simulink model "simulink_stato_scalare"  (R2024a)
settings: Solver=FixedStepAuto  StartTime=0.0  StopTime=T_max  FixedStep=ST  RelTol=1e-3
values from neighbouring files (symbols this model uses):
  a_m = 1    [init.m]
  a_r = 1.1    [init.m]
  alfa = 1    [init.m]
  b_m = 1    [init.m]
  centri_f = zeros(1,numero_nodi_f)    [init.m]
  centri_H = zeros(1,numero_nodi_H)    [init.m]
  k_m = 10    [init.m]
  k_r = 10    [init.m]
  lr_f = 0.2    [init.m]
  lr_H = 1    [init.m]
  M_f = 100    [init.m]
  M_H = 0.5    [init.m]
  numero_nodi_f = 41    [init.m]
  numero_nodi_H = 41    [init.m]
  omega_r = 5*2*pi/T_max    (= 0.261799387799)    [init.m]
  q_init = 0    [init.m]
  q_limit = pi    (= 3.14159265359)    [init.m]
  var_f = delta_q_f^2/2/log(2)    [init.m]
  var_H = delta_q_H^2/2/log(2)    [init.m]
settings Model: Creator=gabri  LastModifiedBy=gabri

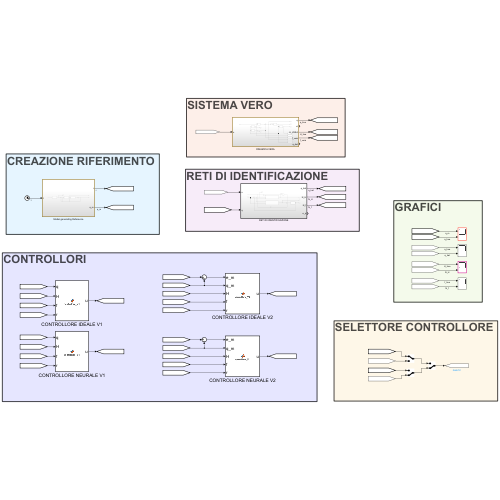
[thumbnail: Simulink's stored preview of the top-level diagram]
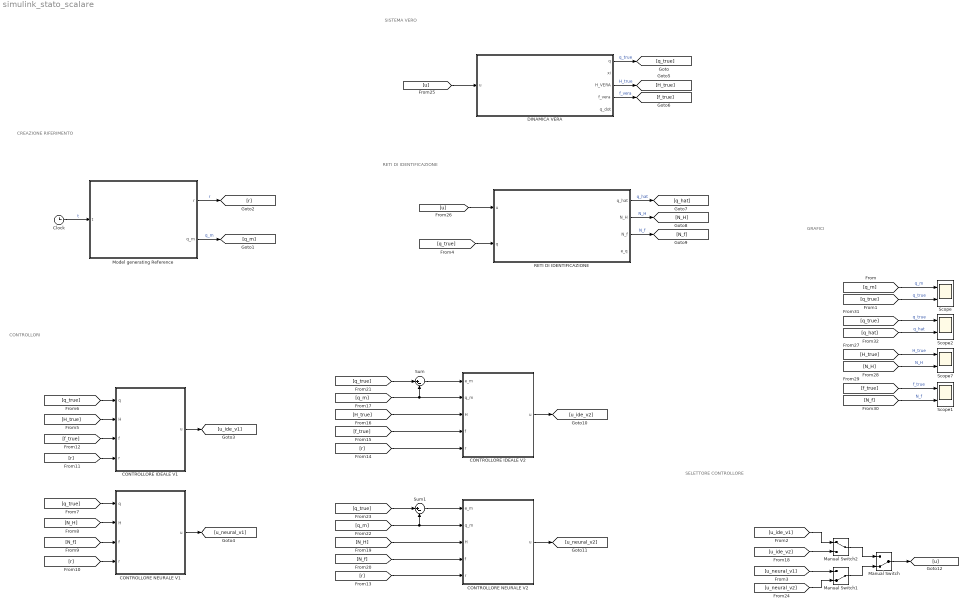
== system simulink_stato_scalare ==
  note: CREAZIONE RIFERIMENTO
  note: RETI DI IDENTIFICAZIONE
  note: SISTEMA VERO
  note: GRAFICI
  note: SELETTORE CONTROLLORE
  note: CONTROLLORI
  CONTROLLORE IDEALE V1 : MATLAB Function  TreatAsAtomicUnit=on
  CONTROLLORE IDEALE V2 : MATLAB Function  TreatAsAtomicUnit=on
  CONTROLLORE NEURALE V1 : MATLAB Function  TreatAsAtomicUnit=on
  CONTROLLORE NEURALE V2 : MATLAB Function  TreatAsAtomicUnit=on
  Clock : Clock
  DINAMICA VERA : Subsystem
  Manual Switch : ManualSwitch  CurrentSetting=0
  Manual Switch1 : ManualSwitch  CurrentSetting=0
  Manual Switch2 : ManualSwitch
  Model generating Reference : Subsystem
  RETI DI IDENTIFICAZIONE : Subsystem
  Scope{,1..2,7} (4 alike) : Scope  NumInputPorts=2
  Sum : Sum  Inputs=|+-
  Sum1 : Sum  Inputs=|+-
  wires:
  Clock/1 -> Model generating Reference/1(t)  "t"
  Model generating Reference/2(q_m) -> [q_m]  "q_m"
  [q_m] -> Scope/1  "q_m"
  [q_true] -> Scope/2  "q_true"
  Model generating Reference/1(r) -> [r]  "r"
  CONTROLLORE IDEALE V1/1(u) -> [u_ide_v1]
  CONTROLLORE NEURALE V1/1(u) -> [u_neural_v1]
  DINAMICA VERA/1(q) -> [q_true]  "q_true"
  DINAMICA VERA/3(H_VERA) -> [H_true]  "H_true"
  DINAMICA VERA/4(f_vera) -> [f_true]  "f_vera"
  Manual Switch1/1 -> Manual Switch/2
  Manual Switch2/1 -> Manual Switch/1
  [u_ide_v1] -> Manual Switch2/1
  [u_neural_v1] -> Manual Switch1/1
  [q_true] -> RETI DI IDENTIFICAZIONE/2(q)
  RETI DI IDENTIFICAZIONE/1(q_hat) -> [q_hat]  "q_hat"
  RETI DI IDENTIFICAZIONE/2(N_H) -> [N_H]  "N_H"
  RETI DI IDENTIFICAZIONE/3(N_f) -> [N_f]  "N_f"
  [H_true] -> CONTROLLORE IDEALE V1/2(H)
  [q_true] -> CONTROLLORE IDEALE V1/1(q)
  [q_true] -> CONTROLLORE NEURALE V1/1(q)
  [N_H] -> CONTROLLORE NEURALE V1/2(H)
  [N_f] -> CONTROLLORE NEURALE V1/3(f)
  [r] -> CONTROLLORE NEURALE V1/4(r)
  [r] -> CONTROLLORE IDEALE V1/4(r)
  [f_true] -> CONTROLLORE IDEALE V1/3(f)
  [f_true] -> CONTROLLORE IDEALE V2/4(f)
  [r] -> CONTROLLORE IDEALE V2/5(r)
  [r] -> CONTROLLORE NEURALE V2/5(r)
  [N_f] -> CONTROLLORE NEURALE V2/4(f)
  [N_H] -> CONTROLLORE NEURALE V2/3(H)
  [q_m] -> Sum/2, CONTROLLORE IDEALE V2/2(q_m)
  [H_true] -> CONTROLLORE IDEALE V2/3(H)
  [q_true] -> Sum/1
  Sum/1 -> CONTROLLORE IDEALE V2/1(e_m)
  Sum1/1 -> CONTROLLORE NEURALE V2/1(e_m)
  [q_true] -> Sum1/1
  [q_m] -> CONTROLLORE NEURALE V2/2(q_m), Sum1/2
  CONTROLLORE NEURALE V2/1(u) -> [u_neural_v2]
  CONTROLLORE IDEALE V2/1(u) -> [u_ide_v2]
  [u_neural_v2] -> Manual Switch1/2
  [u_ide_v2] -> Manual Switch2/2
  Manual Switch/1 -> [u]
  [u] -> DINAMICA VERA/1(u)
  [u] -> RETI DI IDENTIFICAZIONE/1(u)
  [H_true] -> Scope7/1  "H_true"
  [N_H] -> Scope7/2  "N_H"
  [N_f] -> Scope1/2  "N_f"
  [f_true] -> Scope1/1  "f_true"
  [q_hat] -> Scope2/2  "q_hat"
  [q_true] -> Scope2/1  "q_true"

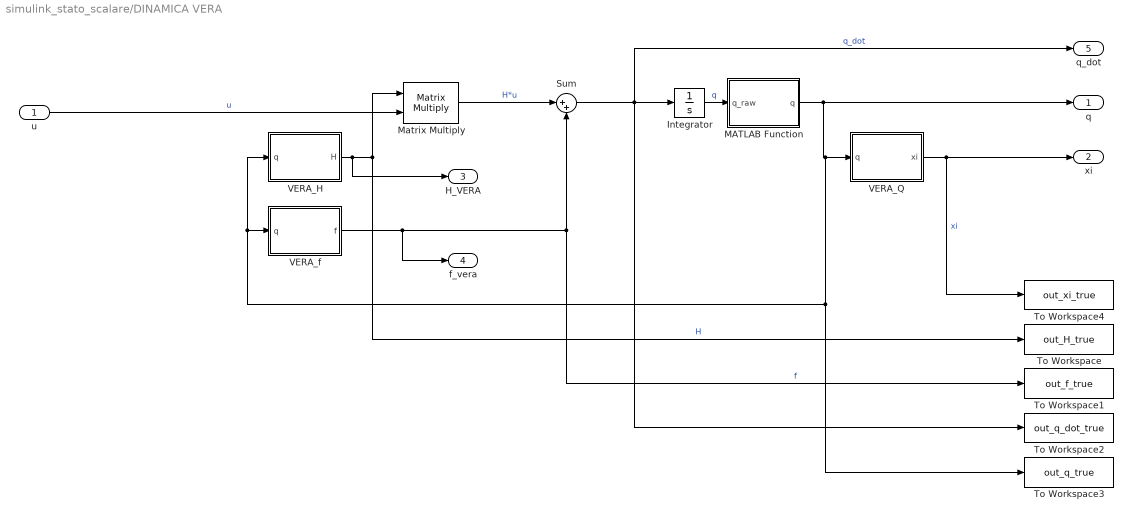
== system simulink_stato_scalare/DINAMICA VERA ==
  u : Inport
  Integrator : Integrator  InitialCondition=q_init
  MATLAB Function : MATLAB Function  TreatAsAtomicUnit=on
  Matrix Multiply : Product  Multiplication=Matrix(*)
  Sum : Sum  Inputs=|++
  To Workspace : ToWorkspace  VariableName=out_H_true  SaveFormat=Timeseries  SampleTime=-1
  To Workspace1 : ToWorkspace  VariableName=out_f_true  SaveFormat=Timeseries  SampleTime=-1
  To Workspace2 : ToWorkspace  VariableName=out_q_dot_true  SaveFormat=Timeseries  SampleTime=-1
  To Workspace3 : ToWorkspace  VariableName=out_q_true  SaveFormat=Timeseries  SampleTime=-1
  To Workspace4 : ToWorkspace  VariableName=out_xi_true  SaveFormat=Timeseries  SampleTime=-1
  VERA_H : MATLAB Function  TreatAsAtomicUnit=on
  VERA_Q : MATLAB Function  TreatAsAtomicUnit=on
  VERA_f : MATLAB Function  TreatAsAtomicUnit=on
  q : Outport
  xi : Outport  Port=2
  H_VERA : Outport  Port=3
  f_vera : Outport  Port=4
  q_dot : Outport  Port=5
  wires:
  VERA_H/1(H) -> H_VERA/1, To Workspace/1, Matrix Multiply/1  "H"
  u/1 -> Matrix Multiply/2  "u"
  Matrix Multiply/1 -> Sum/1  "H*u"
  VERA_f/1(f) -> f_vera/1, To Workspace1/1, Sum/2  "f"
  Sum/1 -> q_dot/1, To Workspace2/1, Integrator/1  "q_dot"
  VERA_Q/1(xi) -> To Workspace4/1, xi/1  "xi"
  Integrator/1 -> MATLAB Function/1(q_raw)  "q"
  MATLAB Function/1(q) -> VERA_H/1(q), VERA_f/1(q), To Workspace3/1, VERA_Q/1(q), q/1

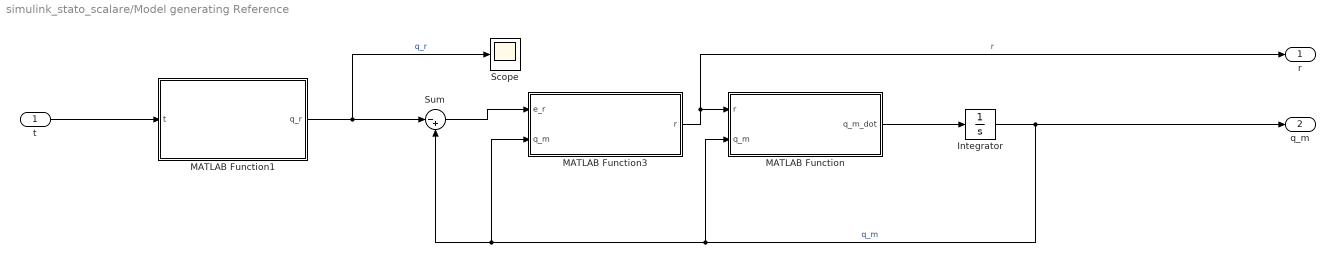
== system simulink_stato_scalare/Model generating Reference ==
  t : Inport
  Integrator : Integrator
  MATLAB Function : MATLAB Function  TreatAsAtomicUnit=on
  MATLAB Function1 : MATLAB Function  TreatAsAtomicUnit=on
  MATLAB Function3 : MATLAB Function  TreatAsAtomicUnit=on
  Scope : Scope
  Sum : Sum  Inputs=|-+
  r : Outport
  q_m : Outport  Port=2
  wires:
  MATLAB Function1/1(q_r) -> Sum/1, Scope/1  "q_r"
  Integrator/1 -> q_m/1, MATLAB Function3/2(q_m), Sum/2, MATLAB Function/2(q_m)  "q_m"
  t/1 -> MATLAB Function1/1(t)
  MATLAB Function3/1(r) -> r/1, MATLAB Function/1(r)  "r"
  MATLAB Function/1(q_m_dot) -> Integrator/1
  Sum/1 -> MATLAB Function3/1(e_r)

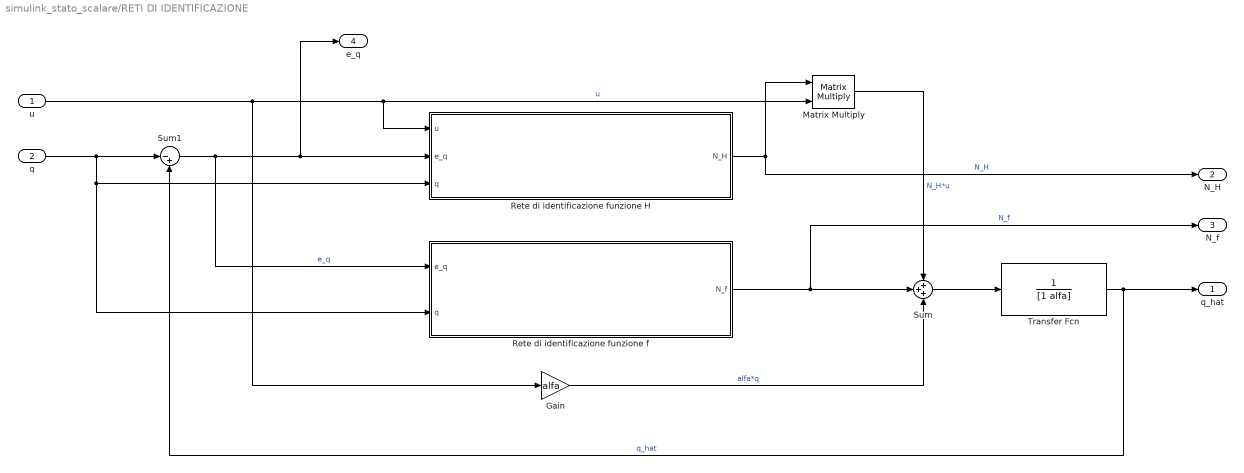
== system simulink_stato_scalare/RETI DI IDENTIFICAZIONE ==
  u : Inport
  q : Inport  Port=2
  Gain : Gain  Gain=alfa
  Matrix Multiply : Product  Multiplication=Matrix(*)
  Rete di identificazione funzione H : Subsystem
  Rete di identificazione funzione f : Subsystem
  Sum : Sum  Inputs=+++
  Sum1 : Sum  Inputs=|-+
  Transfer Fcn : TransferFcn  Denominator=[1 alfa]
  q_hat : Outport
  N_H : Outport  Port=2
  N_f : Outport  Port=3
  e_q : Outport  Port=4
  wires:
  u/1 -> Gain/1, Rete di identificazione funzione H/1(u), Matrix Multiply/2  "u"
  Rete di identificazione funzione H/1(N_H) -> N_H/1, Matrix Multiply/1  "N_H"
  Matrix Multiply/1 -> Sum/1  "N_H*u"
  q/1 -> Sum1/1, Rete di identificazione funzione f/2(q), Rete di identificazione funzione H/3(q)
  Rete di identificazione funzione f/1(N_f) -> N_f/1, Sum/2  "N_f"
  Sum/1 -> Transfer Fcn/1
  Transfer Fcn/1 -> Sum1/2, q_hat/1  "q_hat"
  Gain/1 -> Sum/3  "alfa*q"
  Sum1/1 -> Rete di identificazione funzione f/1(e_q), e_q/1, Rete di identificazione funzione H/2(e_q)  "e_q"

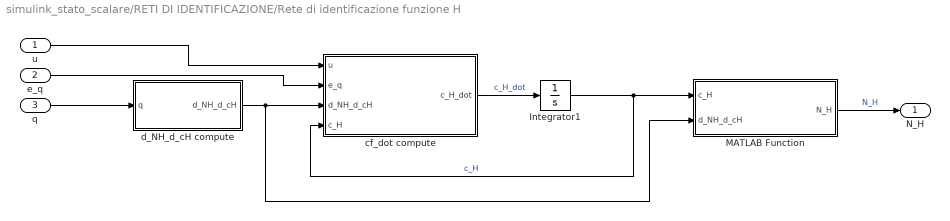
== system simulink_stato_scalare/RETI DI IDENTIFICAZIONE/Rete di identificazione funzione H ==
  u : Inport
  e_q : Inport  Port=2
  q : Inport  Port=3
  Integrator1 : Integrator  InitialCondition=c_H_init'
  MATLAB Function : MATLAB Function  TreatAsAtomicUnit=on
  cf_dot compute : MATLAB Function  TreatAsAtomicUnit=on
  d_NH_d_cH compute : MATLAB Function  TreatAsAtomicUnit=on
  N_H : Outport
  wires:
  MATLAB Function/1(N_H) -> N_H/1  "N_H"
  q/1 -> d_NH_d_cH compute/1(q)
  d_NH_d_cH compute/1(d_NH_d_cH) -> MATLAB Function/2(d_NH_d_cH), cf_dot compute/3(d_NH_d_cH)
  cf_dot compute/1(c_H_dot) -> Integrator1/1  "c_H_dot"
  Integrator1/1 -> MATLAB Function/1(c_H), cf_dot compute/4(c_H)  "c_H"
  e_q/1 -> cf_dot compute/2(e_q)
  u/1 -> cf_dot compute/1(u)

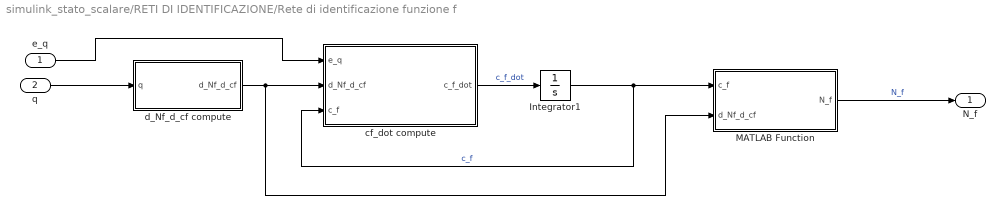
== system simulink_stato_scalare/RETI DI IDENTIFICAZIONE/Rete di identificazione funzione f ==
  e_q : Inport
  q : Inport  Port=2
  Integrator1 : Integrator  InitialCondition=c_f_init'
  MATLAB Function : MATLAB Function  TreatAsAtomicUnit=on
  cf_dot compute : MATLAB Function  TreatAsAtomicUnit=on
  d_Nf_d_cf compute : MATLAB Function  TreatAsAtomicUnit=on
  N_f : Outport
  wires:
  e_q/1 -> cf_dot compute/1(e_q)
  Integrator1/1 -> MATLAB Function/1(c_f), cf_dot compute/3(c_f)  "c_f"
  cf_dot compute/1(c_f_dot) -> Integrator1/1  "c_f_dot"
  d_Nf_d_cf compute/1(d_Nf_d_cf) -> MATLAB Function/2(d_Nf_d_cf), cf_dot compute/2(d_Nf_d_cf)
  q/1 -> d_Nf_d_cf compute/1(q)
  MATLAB Function/1(N_f) -> N_f/1  "N_f"

== matlab function simulink_stato_scalare/Model generating Reference/MATLAB Function ==
  data: r input; q_m_dot output; q_m input; b_m parameter; a_m parameter
function q_m_dot = reference_dynamic(r, q_m, b_m, a_m)

q_m_dot = -a_m*q_m + b_m*r;

== matlab function simulink_stato_scalare/Model generating Reference/MATLAB Function3 ==
  data: e_r input; r output; q_m input; k_r parameter; b_m parameter; a_m parameter
function r = reference_controller(e_r, q_m, k_r, b_m, a_m)

r = (1/b_m)*(a_m*q_m - k_r*e_r);

== matlab function simulink_stato_scalare/CONTROLLORE IDEALE V1 ==
  data: q input; H input; u output; f input; r input; b_m parameter; a_m parameter
function u = controllore_V1(q, H, f, r, b_m, a_m)

u = (1/H)*(-a_m*q + b_m*r - f);

== matlab function simulink_stato_scalare/CONTROLLORE IDEALE V2 ==
  data: e_m input; q_m input; H input; u output; f input; r input; b_m parameter; a_m parameter; k_m parameter
function u = controllore_V2(e_m, q_m, H, f, r, b_m, a_m, k_m)

u = (1/H)*(-a_m*q_m + b_m*r - f -k_m*e_m);

== matlab function simulink_stato_scalare/DINAMICA VERA/VERA_f ==
  data: q input; f output
function f = f(q)

f = (1/2/pi)*sin(2*pi*q);
% f = -q;

== matlab function simulink_stato_scalare/CONTROLLORE NEURALE V2 ==
  data: e_m input; q_m input; H input; u output; f input; r input; b_m parameter; a_m parameter; k_m parameter
function u = controllore_V2(e_m, q_m, H, f, r, b_m, a_m, k_m)

u = (1/H)*(-a_m*q_m + b_m*r - f -k_m*e_m);

== matlab function simulink_stato_scalare/RETI DI IDENTIFICAZIONE/Rete di identificazione funzione H/cf_dot compute ==
  data: u input; e_q input; c_H_dot output; d_NH_d_cH input; M_H parameter; lr_H parameter; c_H input
function c_H_dot = cH_dot(u, e_q, d_NH_d_cH, M_H, lr_H, c_H)

norm_c_H = norm(c_H);

if norm_c_H <= M_H
    c_H_dot = - lr_H * d_NH_d_cH * e_q * u;
else
    c_H_dot = - lr_H * d_NH_d_cH * e_q * u + (lr_H*e_q*c_H'*d_NH_d_cH*u/norm_c_H^2)*c_H;
end

== matlab function simulink_stato_scalare/RETI DI IDENTIFICAZIONE/Rete di identificazione funzione H/d_NH_d_cH compute ==
  data: q input; d_NH_d_cH output; var_H parameter; centri_H parameter; numero_nodi_H parameter
function d_NH_d_cH = d_NH_d_cH(q, var_H, centri_H, numero_nodi_H)

d_NH_d_cH = zeros(numero_nodi_H, 1);

for i=1:numero_nodi_H
    d_NH_d_cH(i) = gaussiana(centri_H(i), var_H, q);
end

== matlab function simulink_stato_scalare/DINAMICA VERA/VERA_H ==
  data: q input; H output
function H = H(q)

H = 1+(1/5/pi)*cos(5*pi*q);
% H = 1;

== matlab function simulink_stato_scalare/DINAMICA VERA/MATLAB Function ==
  data: q_raw input; q output
function q = wrap_to_pi(q_raw)

q = atan2(sin(q_raw), cos(q_raw));

== matlab function simulink_stato_scalare/DINAMICA VERA/VERA_Q ==
  data: q input; xi output
function xi = Q(q)

xi = 10*cos(q);

== matlab function simulink_stato_scalare/RETI DI IDENTIFICAZIONE/Rete di identificazione funzione f/MATLAB Function ==
  data: c_f input; N_f output; d_Nf_d_cf input
function N_f = N_f(c_f, d_Nf_d_cf)

N_f = c_f'*d_Nf_d_cf;

== matlab function simulink_stato_scalare/RETI DI IDENTIFICAZIONE/Rete di identificazione funzione H/MATLAB Function ==
  data: c_H input; N_H output; d_NH_d_cH input
function N_H = N_H(c_H, d_NH_d_cH)

N_H = (0.5*ones(1, length(c_H)) + c_H')*d_NH_d_cH;

== matlab function simulink_stato_scalare/RETI DI IDENTIFICAZIONE/Rete di identificazione funzione f/d_Nf_d_cf compute ==
  data: q input; d_Nf_d_cf output; var_f parameter; centri_f parameter; numero_nodi_f parameter
function d_Nf_d_cf = d_Nf_d_cf(q, var_f, centri_f, numero_nodi_f)

d_Nf_d_cf = zeros(numero_nodi_f, 1);

for i=1:numero_nodi_f
    d_Nf_d_cf(i,1) = gaussiana(centri_f(i), var_f, q);
end

== matlab function simulink_stato_scalare/RETI DI IDENTIFICAZIONE/Rete di identificazione funzione f/cf_dot compute ==
  data: e_q input; c_f_dot output; d_Nf_d_cf input; c_f input; M_f parameter; lr_f parameter
function c_f_dot = cf_dot(e_q, d_Nf_d_cf, c_f, M_f, lr_f)

norm_c_f = norm(c_f);

if norm_c_f <= M_f
    c_f_dot = - lr_f * d_Nf_d_cf * e_q;
else
    c_f_dot = - lr_f * d_Nf_d_cf * e_q + (lr_f*e_q*c_f'*d_Nf_d_cf/norm_c_f^2)*c_f;
end

== matlab function simulink_stato_scalare/Model generating Reference/MATLAB Function1 ==
  data: t input; q_r output; q_limit parameter; omega_r parameter; a_r parameter
function q_r  = q_ref(t, q_limit, omega_r, a_r)

q_r = (q_limit/2)*(sin(a_r*omega_r*t) + sin((1+a_r)*omega_r*t));

== matlab function simulink_stato_scalare/CONTROLLORE NEURALE V1 ==
  data: q input; H input; u output; f input; r input; b_m parameter; a_m parameter
function u = controllore_V1(q, H, f, r, b_m, a_m)

u = (1/H)*(-a_m*q + b_m*r - f);
